simulink model "Aircraft_GNC"  (R2021b)
settings: Solver=FixedStepAuto  StartTime=0.0  StopTime=45  RelTol=1e-3
values from neighbouring files (symbols this model uses):
  A = [-1.064 1; 290.26 0]    [GNC_aircraft.m]
  B = [-0.25; -331.40]    [GNC_aircraft.m]
  C = [-123.34 0; 0 1]    [GNC_aircraft.m]
  D = [-13.51; 0]    [GNC_aircraft.m]
  dT1 = 0.75    [GNC_aircraft.m]
  dT2 = 0.25    [GNC_aircraft.m]
  ELEV_INIT = 3267    [GNC_aircraft.m]
  ELEV_TARGET = 402    [GNC_aircraft.m]
  LAT_INIT = 46.8267    [GNC_aircraft.m]
  LAT_OBST = 46.9383    [GNC_aircraft.m]
  LAT_TARGET = 47.2235    [GNC_aircraft.m]
  LONG_INIT = 8.8286    [GNC_aircraft.m]
  LONG_OBST = 8.7508    [GNC_aircraft.m]
  LONG_TARGET = 8.7190    (= 8.719)    [GNC_aircraft.m]
  vel = 1021.08    [GNC_aircraft.m]
undefined symbols (not defined in the file or in its folder): Earth, K, L, WGS84
libraries: simulink x3, aerolibfltsims x2, slpidlib x1, aerolibtransform2 x1
settings Model: Creator=hashi  LastModifiedBy=hashi

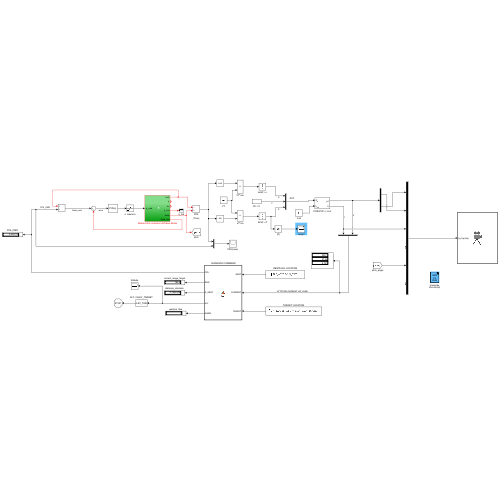
[thumbnail: Simulink's stored preview of the top-level diagram]
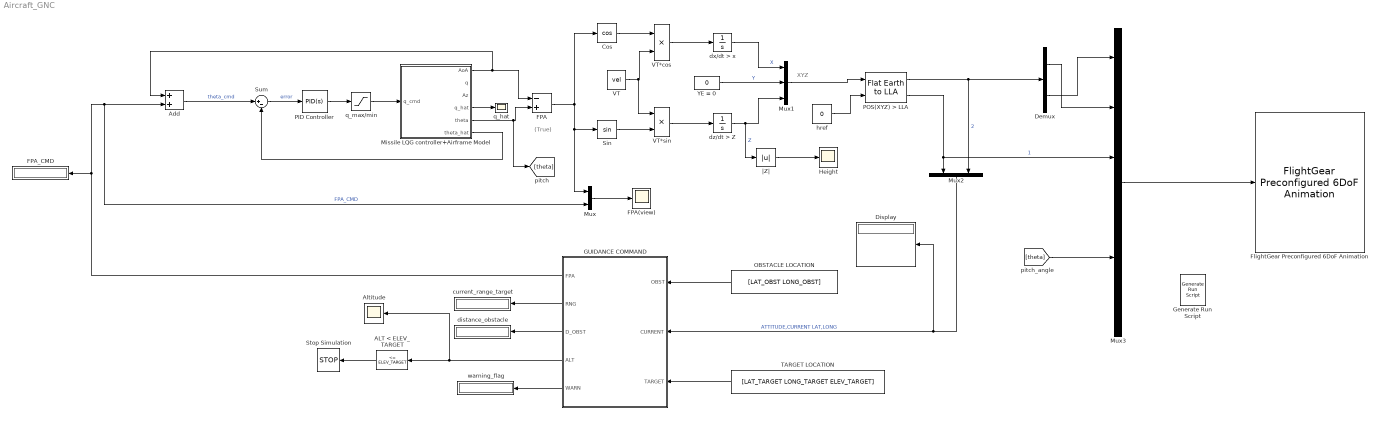
== system Aircraft_GNC ==
  note: XYZ
  note: (True)
  " ALT < ELEV_TARGET" : simulink/Logic and Bit Operations/Compare To Constant  relop=<=  const=ELEV_TARGET  OutDataTypeStr=boolean
  " GUIDANCE COMMAND" : MATLAB Function  TreatAsAtomicUnit=on
  Add : Sum
  Altitude : Scope
  Cos : Trigonometry  Operator=cos
  Demux : Demux  Outputs=2
  Display : Display
      settings: Decimation=3
  FPA : Sum  Inputs=-+
  FPA(view) : Scope
  FPA_CMD : Display
  FlightGear Preconfigured 6DoF Animation : aerolibfltsims/FlightGear Preconfigured 6DoF Animation  xFlightGearVersion=v2019.1  DestinationIpAddress=127.0.0.1  DestinationPort=5502  SampleTime=1/30  packetVersion=24
  Generate Run Script : aerolibfltsims/Generate Run Script  Architecture=Win64  dataFlow=Send  GeometryModelName=lightning  AirportId=KSFO  RunwayId=10L  InitialAltitude=7224  InitialHeading=113  OffsetDistance=4.72  OffsetAzimuth=0  InstallScenery=on  DisableShaders=on  OriginAddress=127.0.0.1  DestinationPort=5502  OriginPort=5505  LocalAddress=127.0.0.1  OutputFileName=runfg.bat  FlightGearBaseDirectory=C:\Program Files\FlightGear 2020.3
  Height : Scope
  Missile LQG controller+Airframe Model : Subsystem
  Mux : Mux  Inputs=2
  Mux1 : Mux  Inputs=3
  Mux2 : Mux  Inputs=2
  Mux3 : Mux  Inputs=6
  OBSTACLE LOCATION : Constant  Value=[LAT_OBST LONG_OBST]
  PID Controller : slpidlib/PID Controller  Controller=PID  Form=Parallel  TimeDomain=Continuous-time  UseExternalTs=off  SampleTime=-1  IntegratorMethod=Forward Euler  FilterMethod=Forward Euler  ControllerParametersSource=internal  P=-1  I=0  D=0  UseFilter=on  N=100  TunerSelectOption=Transfer Function Based (PID Tuner App)  InitialConditionSource=internal  InitialConditionForIntegrator=0  InitialConditionForFilter=0  DifferentiatorICPrevScaledInput=0  ExternalReset=none  TrackingMode=off  Kt=1  LimitOutput=off  SatLimitsSource=internal  UpperSaturationLimit=inf  LowerSaturationLimit=-inf  LinearizeAsGain=on  AntiWindupMode=none  Kb=1  POutMin=[]  POutMax=[]  IOutMin=[]  IOutMax=[]  DOutMin=[]  DOutMax=[]  NOutMin=[]  NOutMax=[]  SumOutMin=[]  SumOutMax=[]  SaturationOutMin=[]  SaturationOutMax=[]  PParamMin=[]  PParamMax=[]  IParamMin=[]  IParamMax=[]  DParamMin=[]  DParamMax=[]  NParamMin=[]  NParamMax=[]  KbParamMin=[]  KbParamMax=[]  KtParamMin=[]  KtParamMax=[]  KbOutMin=[]  KbOutMax=[]  KtOutMin=[]  KtOutMax=[]  IntegratorOutMin=[]  IntegratorOutMax=[]  FilterOutMin=[]  FilterOutMax=[]  SumI1OutMin=[]  SumI1OutMax=[]  SumI2OutMin=[]  SumI2OutMax=[]  SumI3OutMin=[]  SumI3OutMax=[]  SumI4OutMin=[]  SumI4OutMax=[]  SumDOutMin=[]  SumDOutMax=[]  DifferentiatorOutMin=[]  DifferentiatorOutMax=[]  FilterDiffOutCoefMin=[]  FilterDiffOutCoefMax=[]  ReciprocalOutMin=[]  ReciprocalOutMax=[]  SumDenOutMin=[]  SumDenOutMax=[]  SumNumOutMin=[]  SumNumOutMax=[]  DivideOutMin=[]  DivideOutMax=[]  UdiffTsProdOutMin=[]  UdiffTsProdOutMax=[]  NTsProdOutMin=[]  NTsProdOutMax=[]  UintegralTsProdOutMin=[]  UintegralTsProdOutMax=[]  UngainTsProdOutMin=[]  UngainTsProdOutMax=[]  IntegratorContinuousStateAttributes=''  IntegratorStateMustResolveToSignalObject=off  IntegratorRTWStateStorageClass=Auto  FilterContinuousStateAttributes=''  FilterStateMustResolveToSignalObject=off  FilterRTWStateStorageClass=Auto  ParallelPVariant=InternalParameters  IdealPVariant=Disabled  IVariant=InternalParameters  DVariant=InternalParameters  IntegratorVariant=Continuous  SatVariant=Disabled  AWVariant=Passthrough  PCopyVariant=Disabled  TRVariant=Disabled  FdbkBlocksVariant=Forward  IdealPFdbkVariant=Disabled  SatFdbkVariant=Disabled  DerivativeFilterVariant=ContFilter  NVariant=InternalParameters  NCopyVariant=Disabled  FilterICVariant=InternalICsFilter  IntegratorICVariant=InternalICs  ExternalResetVariant=Disabled  TRSumVariant=Passthrough  SumFdbkVariant=Disabled  SumVariant=Sum_PID  TsampFilterVariant=InternalTs  TsampNgainVariant=Passthrough  TsampIntegralVariant=Passthrough  ExternalSaturationOutDataTypeStr=Inherit: Same as second input
  POS(XYZ) > LLA : aerolibtransform2/Flat Earth to LLA  units=Metric (MKS)  ptype=Earth (WGS84)  F=1/298.257223563  R=6378137  refPosPort=off  LL0=[LAT_INIT LONG_INIT]  psi=yaw_init
  Sin : Trigonometry
  Stop Simulation : Stop
  Sum : Sum  Inputs=|+-
  TARGET LOCATION : Constant  Value=[LAT_TARGET LONG_TARGET ELEV_TARGET]
  VT : Constant  Value=vel
  VT*cos : Product
  VT*sin : Product
  "YE = 0 " : Constant  Value=0
  current_range_target : Display
  distance_obstacle : Display
  dx/dt > x : Integrator
  dz/dt > Z : Integrator  InitialCondition=-ELEV_INIT
  href : Constant  Value=0
  q_hat : Scope
  q_max/min : Saturate
  warning_flag : Display
  |Z| : Abs
  wires:
  PID Controller/1 -> q_max/min/1
  q_max/min/1 -> Missile LQG controller+Airframe Model/1(" q_cmd")
  Sum/1 -> PID Controller/1  "error"
  Add/1 -> Sum/1  "theta_cmd"
  Missile LQG controller+Airframe Model/6(theta_hat) -> Sum/2
  Missile LQG controller+Airframe Model/1(AoA) -> FPA/1, Add/1
  Missile LQG controller+Airframe Model/5(theta) -> [theta], FPA/2
  " GUIDANCE COMMAND"/1(FPA) -> FPA_CMD/1, Mux/2, Add/2  "FPA_CMD"
  FPA/1 -> Mux/1, Sin/1, Cos/1
  Mux/1 -> FPA(view)/1
  Cos/1 -> VT*cos/1
  Sin/1 -> VT*sin/2
  VT/1 -> VT*sin/1, VT*cos/2
  VT*sin/1 -> dz/dt > Z/1
  VT*cos/1 -> dx/dt > x/1
  dx/dt > x/1 -> Mux1/1  "X"
  "YE = 0 "/1 -> Mux1/2  "Y"
  dz/dt > Z/1 -> |Z|/1, Mux1/3  "Z"
  Missile LQG controller+Airframe Model/4(q_hat) -> q_hat/1
  |Z|/1 -> Height/1
  href/1 -> POS(XYZ) > LLA/2
  Mux1/1 -> POS(XYZ) > LLA/1
  POS(XYZ) > LLA/2 -> Mux3/3, Mux2/1  "1"
  POS(XYZ) > LLA/1 -> Demux/1, Mux2/2  "2"
  OBSTACLE LOCATION/1 -> " GUIDANCE COMMAND"/1(OBST)
  TARGET LOCATION/1 -> " GUIDANCE COMMAND"/3(TARGET)
  Mux2/1 -> Display/1, " GUIDANCE COMMAND"/2(CURRENT)  "ATTITUDE,CURRENT LAT,LONG"
  " GUIDANCE COMMAND"/2(RNG) -> current_range_target/1
  " GUIDANCE COMMAND"/3(D_OBST) -> distance_obstacle/1
  " GUIDANCE COMMAND"/5(WARN) -> warning_flag/1
  " ALT < ELEV_TARGET"/1 -> Stop Simulation/1
  " GUIDANCE COMMAND"/4(ALT) -> Altitude/1, " ALT < ELEV_TARGET"/1
  Mux3/1 -> FlightGear Preconfigured 6DoF Animation/1
  Demux/2 -> Mux3/1
  Demux/1 -> Mux3/2
  [theta] -> Mux3/5

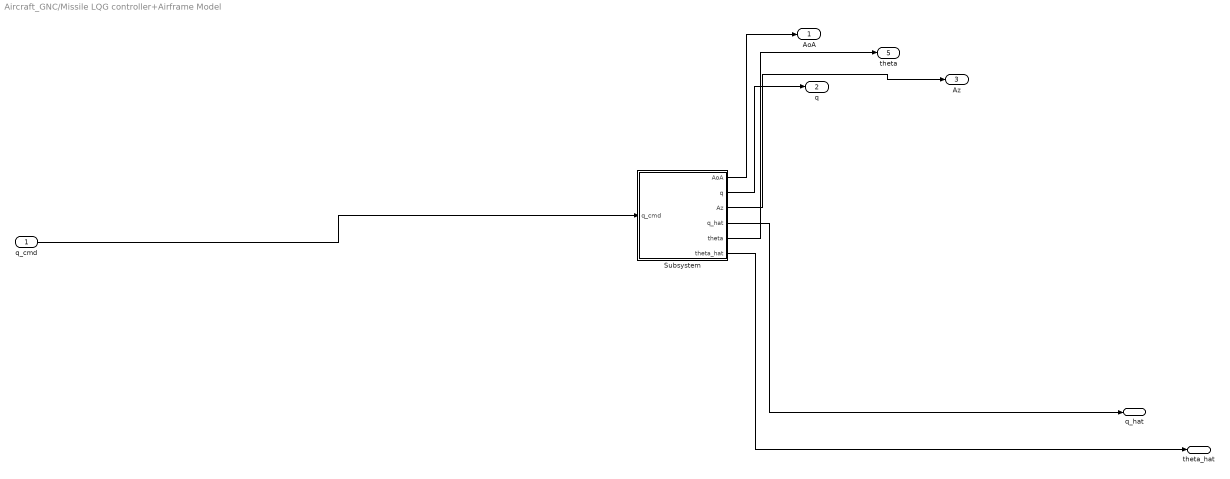
== system Aircraft_GNC/Missile LQG controller+Airframe Model ==
  " q_cmd" : Inport
  Subsystem : Subsystem
  AoA : Outport
  q : Outport  Port=2
  Az : Outport  Port=3
  q_hat : Outport  Port=4
  theta : Outport  Port=5
  theta_hat : Outport  Port=6
  wires:
  Subsystem/4(q_hat) -> q_hat/1
  Subsystem/1(AoA) -> AoA/1
  Subsystem/3(Az) -> Az/1
  Subsystem/2(q) -> q/1
  Subsystem/6(theta_hat) -> theta_hat/1
  " q_cmd"/1 -> Subsystem/1(" q_cmd")
  Subsystem/5(theta) -> theta/1

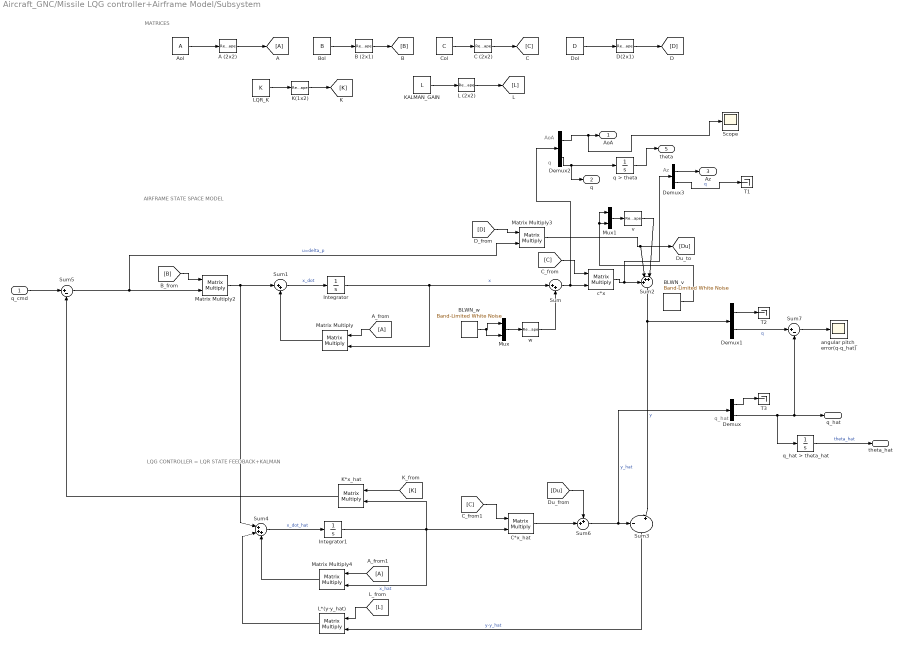
== system Aircraft_GNC/Missile LQG controller+Airframe Model/Subsystem ==
  note: Az
  note: AoA
  note: q
  note: q_hat
  note: LQG CONTROLLER = LQR STATE FEEDBACK+KALMAN
  note: AIRFRAME STATE SPACE MODEL
  note: MATRICES
  " q_cmd" : Inport
  " C*x_hat" : Product  Multiplication=Matrix(*)
  A (2x2) : Reshape  OutputDimensionality=Customize  OutputDimensions=[2,2]
  Aol : Constant  Value=A
  B (2x1) : Reshape  OutputDimensionality=Customize  OutputDimensions=[2,1]
  BLWN_v : simulink/Sources/Band-Limited White Noise  Cov=[0.00001]  Ts=dT2  seed=[23341]
  BLWN_w : simulink/Sources/Band-Limited White Noise  Cov=[0.00000001]  Ts=dT1  seed=[23341]
  Bol : Constant  Value=B
  C (2x2) : Reshape  OutputDimensionality=Customize  OutputDimensions=[2,2]
  Col : Constant  Value=C
  D(2x1) : Reshape  OutputDimensionality=Customize  OutputDimensions=[2,1]
  Demux{,1..3} (4 alike) : Demux  Outputs=2
  Dol : Constant  Value=D
  Integrator : Integrator
  Integrator1 : Integrator
  K(1x2) : Reshape  OutputDimensionality=Customize  OutputDimensions=[1,2]
  K*x_hat : Product  Multiplication=Matrix(*)
  KALMAN_GAIN : Constant  Value=L
  L (2x2) : Reshape  OutputDimensionality=Customize  OutputDimensions=[2,2]
  L*(y-y_hat) : Product  Multiplication=Matrix(*)
  LQR_K : Constant  Value=K
  Matrix Multiply{,2..4} (4 alike) : Product  Multiplication=Matrix(*)
  Mux : Mux  Inputs=2
  Mux1 : Mux  Inputs=2
  Scope : Scope
  Sum : Sum  Inputs=|++
  Sum1 : Sum  Inputs=|++
  Sum2 : Sum  Inputs=+++|
  Sum3 : Sum  Inputs=-|+|
  Sum4 : Sum  Inputs=|+++
  Sum5 : Sum  Inputs=|+-
  Sum6 : Sum  Inputs=++|
  Sum7 : Sum  Inputs=|+-
  T1 : Terminator
  T2 : Terminator
  T3 : Terminator
  angular pitch_error(q-q_hat) : Scope
  c*x : Product  Multiplication=Matrix(*)
  q > theta : Integrator
  q_hat > theta_hat : Integrator
  v : Reshape  OutputDimensionality=Customize  OutputDimensions=[2,1]
  w : Reshape  OutputDimensionality=Customize  OutputDimensions=[2,1]
  AoA : Outport
  q : Outport  Port=2
  Az : Outport  Port=3
  q_hat : Outport  Port=4
  theta : Outport  Port=5
  theta_hat : Outport  Port=6
  wires:
  BLWN_w/1 -> Mux/2, Mux/1
  [L] -> L*(y-y_hat)/1
  " q_cmd"/1 -> Sum5/1
  Demux/1 -> T3/1
  Sum4/1 -> Integrator1/1  "x_dot_hat"
  K*x_hat/1 -> Sum5/2
  Mux/1 -> w/1
  [A] -> Matrix Multiply/1
  Demux1/2 -> Sum7/1  "q"
  Demux3/1 -> Az/1
  q_hat > theta_hat/1 -> theta_hat/1  "theta_hat"
  Demux3/2 -> T1/1  "q"
  Demux1/1 -> T2/1
  Sum5/1 -> Matrix Multiply3/2, Matrix Multiply2/2  "u=delta_p"
  BLWN_v/1 -> Mux1/1, Mux1/2
  Sum1/1 -> Integrator/1  "x_dot"
  Sum2/1 -> Sum3/2, Demux1/1  "y"
  Aol/1 -> A (2x2)/1
  Integrator1/1 -> K*x_hat/2, Matrix Multiply4/2, " C*x_hat"/2  "x_hat"
  Matrix Multiply3/1 -> [Du], Sum2/2
  A (2x2)/1 -> [A]
  Integrator/1 -> Sum/1, Matrix Multiply/2  "x"
  [C] -> " C*x_hat"/1
  Sum3/1 -> L*(y-y_hat)/2  "y-y_hat"
  [A] -> Matrix Multiply4/1
  Sum/1 -> Demux2/1, c*x/2
  Demux2/1 -> Scope/1, AoA/1
  Demux/2 -> q_hat > theta_hat/1, q_hat/1, Sum7/2
  Sum7/1 -> angular pitch_error(q-q_hat)/1
  Matrix Multiply/1 -> Sum1/2
  C (2x2)/1 -> [C]
  L*(y-y_hat)/1 -> Sum4/2
  " C*x_hat"/1 -> Sum6/2
  c*x/1 -> Demux3/1, Sum2/1
  Col/1 -> C (2x2)/1
  KALMAN_GAIN/1 -> L (2x2)/1
  [B] -> Matrix Multiply2/1
  LQR_K/1 -> K(1x2)/1
  [D] -> Matrix Multiply3/1
  Demux2/2 -> q > theta/1, q/1
  Mux1/1 -> v/1
  B (2x1)/1 -> [B]
  q > theta/1 -> theta/1
  Sum6/1 -> Demux/1, Sum3/1  "y_hat"
  [Du] -> Sum6/1
  [K] -> K*x_hat/1
  v/1 -> Sum2/3
  Bol/1 -> B (2x1)/1
  w/1 -> Sum/2
  K(1x2)/1 -> [K]
  [C] -> c*x/1
  Matrix Multiply2/1 -> Sum1/1, Sum4/1
  Matrix Multiply4/1 -> Sum4/3
  Dol/1 -> D(2x1)/1
  D(2x1)/1 -> [D]
  L (2x2)/1 -> [L]

== matlab function Aircraft_GNC/ GUIDANCE COMMAND ==
  data: OBST input; FPA output; CURRENT input; TARGET input; RNG output; D_OBST output; ALT output; WARN output
function [FPA, RNG,D_OBST,ALT,WARN] = fcn(OBST, CURRENT, TARGET)

R = 6371e3; % Earth radius in meters

%OBSTACLE LOCATION
LAT_OBST = OBST(1);
LONG_OBST = OBST(2);


%OBSTACLE THRESHOLD (ZONE)
thresh = 4000; %1km


%TARGET LOCATION
LAT_TARGET= TARGET(1);
LONG_TARGET= TARGET(2);
ELEV_TARGET = TARGET(3);% m-MSL

%CURRENT LOCATION
ELEV_CUR = CURRENT(1);
LAT_CUR = CURRENT(2);
LONG_CUR = CURRENT(3);

%% DISTANCE TO THE TARGET
%here use haversine formula to find the distance from curr to target.
l1 = deg_rad(LAT_CUR);
u1 = deg_rad(LONG_CUR);
l2 = deg_rad(LAT_TARGET);
u2 = deg_rad(LONG_TARGET);
dh = abs(ELEV_TARGET-ELEV_CUR);

delta_l = l2-l1;
delta_u = u2-u1;

h = sin(delta_l/2)^2 + cos(l1)*cos(l2)*sin(delta_u/2)^2;
a = 2*atan2(sqrt(h),sqrt(1-h));
d = R*a


%% DISTANCE FROM THE OBSTACLE
l3 = deg_rad(LAT_OBST);
u3 = deg_rad(LONG_OBST);

%dh_obs = abs(ELEV_OBST-ELEV_CUR);

delta_l = l3-l1;
delta_u = u3-u1;

h = sin(delta_l/2)^2 + cos(l1)*cos(l2)*sin(delta_u/2)^2;
a = 2*atan2(sqrt(h),sqrt(1-h));
d_obst = R*a

%% CURRENT RANGE (from target) -- RANGE > DISTANCE
range = sqrt(d^2 + dh^2);

%% CALCULATE COMMANDED FLIGHT PATH SETPOINT BASED ON D_OBST, RANGE

if abs(d_obst)>=thresh
    flag = 0;
    FPA_CMD = atan(dh/d);
else
    %when in the obstacle zone area, initiate warning signal
    flag = 1;
    FPA_CMD = 0;
end    

%% OUTPUT VARIABLES
FPA = FPA_CMD;
RNG = range;
D_OBST= d_obst;
WARN = flag;
ALT = ELEV_CUR;
